simulink model "Regulator_o_zmiennej_strukturze1"  (R2015a)
settings: Solver=ode3  StartTime=0.0  StopTime=50  FixedStep=0.01  RelTol=1e-3
libraries: simulink x2
settings Model: Creator=lenovo  LastModifiedBy=lenovo

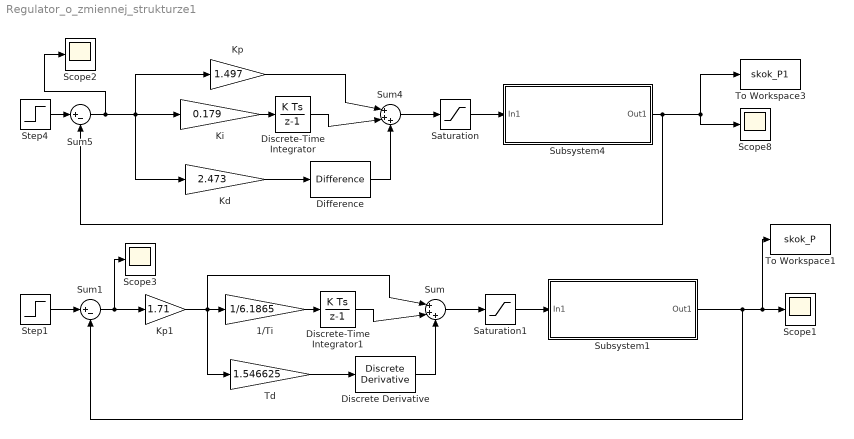
== system Regulator_o_zmiennej_strukturze1 ==
  1/Ti : Gain  Gain=1/6.1865
  Difference : simulink/Discrete/Difference  ICPrevInput=0.0  InputProcessing=Inherited  OutMin=[]  OutMax=[]  OutDataType=fixdt(1, 16)  OutScaling=2^-10  DoSatur=off
  Discrete Derivative : simulink/Discrete/Discrete Derivative  gainval=1.0  ICPrevScaledInput=0.0  InputProcessing=Inherited  OutMin=[]  OutMax=[]  OutDataType=fixdt(1, 16)  OutScaling=2^-10  DoSatur=off
  Discrete-Time Integrator : DiscreteIntegrator  InitialConditionSetting=State (most efficient)  SampleTime=0.01
  Discrete-Time Integrator1 : DiscreteIntegrator  InitialConditionSetting=State (most efficient)  SampleTime=0.01
  Kd : Gain  Gain=2.473
  Ki : Gain  Gain=0.179
  Kp : Gain  Gain=1.497
  Kp1 : Gain  Gain=1.71
  Saturation : Saturate  UpperLimit=1.05  LowerLimit=.9
  Saturation1 : Saturate  UpperLimit=1.3  LowerLimit=-.2
  Scope{1..3,8} (4 alike) : Scope
      Scope1 settings: TimeRange=50  YMin=0.5811999999996471  YMax=0.581199999999775
      Scope2 settings: TimeRange=50  YMin=0.5811999999996471  YMax=0.581199999999775
      Scope3 settings: TimeRange=50  YMin=0.5811999999996471  YMax=0.581199999999775  SaveName=ScopeData2
      Scope8 settings: TimeRange=50  YMin=0.5811999999996471  YMax=0.581199999999775  SaveName=ScopeData7
  Step1 : Step  SampleTime=0
  Step4 : Step  SampleTime=0
  Subsystem1 : Subsystem
  Subsystem4 : Subsystem
  Sum : Sum  Inputs=|+++
  Sum1 : Sum  Inputs=|+-
  Sum4 : Sum  Inputs=|+++
  Sum5 : Sum  Inputs=|+-
  Td : Gain  Gain=1.546625
  To Workspace1 : ToWorkspace  VariableName=skok_P  SaveFormat=Timeseries  SampleTime=-1
  To Workspace3 : ToWorkspace  VariableName=skok_P1  SaveFormat=Timeseries  SampleTime=-1
  wires:
  Ki/1 -> Discrete-Time Integrator/1
  Kd/1 -> Difference/1
  Sum4/1 -> Saturation/1
  Saturation/1 -> Subsystem4/1(In1)
  Difference/1 -> Sum4/3
  Discrete-Time Integrator/1 -> Sum4/2
  Kp/1 -> Sum4/1
  Sum5/1 -> Scope2/1, Kd/1, Kp/1, Ki/1
  Subsystem4/1(Out1) -> Sum5/2, To Workspace3/1, Scope8/1
  Step4/1 -> Sum5/1
  Sum1/1 -> Scope3/1, Kp1/1
  1/Ti/1 -> Discrete-Time Integrator1/1
  Kp1/1 -> Td/1, Sum/1, 1/Ti/1
  Td/1 -> Discrete Derivative/1
  Sum/1 -> Saturation1/1
  Discrete Derivative/1 -> Sum/3
  Discrete-Time Integrator1/1 -> Sum/2
  Saturation1/1 -> Subsystem1/1(In1)
  Subsystem1/1(Out1) -> Sum1/2, To Workspace1/1, Scope1/1
  Step1/1 -> Sum1/1

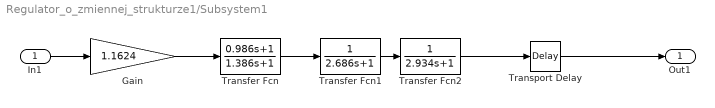
== system Regulator_o_zmiennej_strukturze1/Subsystem1 ==
  In1 : Inport
  Gain : Gain  Gain=1.1624
  Transfer Fcn : TransferFcn  Numerator=[0.986 1]  Denominator=[1.386 1]
  Transfer Fcn1 : TransferFcn  Denominator=[2.686 1]
  Transfer Fcn2 : TransferFcn  Denominator=[2.934 1]
  Transport Delay : TransportDelay  DelayTime=2.122  BufferSize=21504
  Out1 : Outport
  wires:
  Transfer Fcn1/1 -> Transfer Fcn2/1
  Transfer Fcn/1 -> Transfer Fcn1/1
  Transfer Fcn2/1 -> Transport Delay/1
  Transport Delay/1 -> Out1/1
  Gain/1 -> Transfer Fcn/1
  In1/1 -> Gain/1

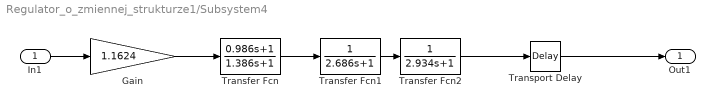
== system Regulator_o_zmiennej_strukturze1/Subsystem4 ==
  In1 : Inport
  Gain : Gain  Gain=1.1624
  Transfer Fcn : TransferFcn  Numerator=[0.986 1]  Denominator=[1.386 1]
  Transfer Fcn1 : TransferFcn  Denominator=[2.686 1]
  Transfer Fcn2 : TransferFcn  Denominator=[2.934 1]
  Transport Delay : TransportDelay  DelayTime=2.122  BufferSize=21504
  Out1 : Outport
  wires:
  Transfer Fcn1/1 -> Transfer Fcn2/1
  Transfer Fcn/1 -> Transfer Fcn1/1
  Transfer Fcn2/1 -> Transport Delay/1
  Transport Delay/1 -> Out1/1
  Gain/1 -> Transfer Fcn/1
  In1/1 -> Gain/1
